simulink model "lab01z3_sch"  (R2021a)
settings: Solver=VariableStepAuto  StartTime=0.0  StopTime=10.0  RelTol=1e-3
InitFcn:
  | close all; clear all; clc;
  | % Parametry obiektu
  | R = 0.2; % [Omega]
  | L = 0.1; % [H]
  | kfi = 0.15; % [Nm/A]
  | m = 2; % [kg]
  | r = 0.2; % [m]
  | b = 0.4 % [Nm/s]
  | g = 9.81; % [m/s^2]
settings Model: Creator=user  LastModifiedBy=AgraWoodAdmin
settings SolverCC: AlgebraicLoopSolver=TrustRegion
settings DataIOCC: ReturnWorkspaceOutputs=off
settings DebuggingCC: SFMachineParentedDataDiag=warning  ArithmeticOperatorsInVariantConditions=warning
settings SFSimCC: SimUseLocalCustomCode=off  CustomCodeUndefinedFunction=UseInterfaceOnly
settings RTWCC: RTWUseLocalCustomCode=off

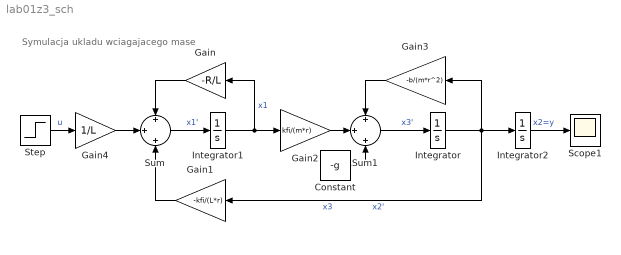
== system lab01z3_sch ==
  note: Symulacja ukladu wciagajacego mase
  Constant : Constant  Value=-g
  Gain : Gain  Gain=-R/L
  Gain1 : Gain  Gain=-kfi/(L*r)
  Gain2 : Gain  Gain=kfi/(m*r)
  Gain3 : Gain  Gain=-b/(m*r^2)
  Gain4 : Gain  Gain=1/L
  Integrator : Integrator
  Integrator1 : Integrator
  Integrator2 : Integrator
  Scope1 : Scope
  Step : Step  Time=0  After=10  SampleTime=0
  Sum : Sum  Inputs=+|+|+
  Sum1 : Sum  Inputs=+|+|+
  wires:
  Step/1 -> Gain4/1  "u"
  Gain4/1 -> Sum/2
  Sum/1 -> Integrator1/1  "x1'"
  Integrator1/1 -> Gain2/1, Gain/1  "x1"
  Gain/1 -> Sum/1
  Gain2/1 -> Sum1/2
  Gain3/1 -> Sum1/1
  Sum1/1 -> Integrator/1  "x3'"
  Integrator/1 -> Integrator2/1, Gain1/1, Gain3/1  "x3               x2'"
  Gain1/1 -> Sum/3
  Integrator2/1 -> Scope1/1  "x2=y"
  Constant/1 -> Sum1/3
